simulink model "adaptive_control"  (R2019a)
settings: Solver=ode3  StartTime=0.0  StopTime=15  FixedStep=.002  RelTol=1e-3  EnableMultiTasking=on
settings Model: ExtModeTrigDuration=10000  Creator=smascaro  LastModifiedBy=hoops
settings SolverCC: PositivePriorityOrder=on
settings DataIOCC: SaveFormat=Array  SignalLoggingSaveFormat=ModelDataLogs  SaveOutput=off  SaveTime=off  ReturnWorkspaceOutputs=off
settings OptimizationCC: ExpressionDepthLimit=2147483647  InitFltsAndDblsToZero=on  LifeSpan=inf
settings DebuggingCC: SaveWithParameterizedLinksMsg=none  UnderspecifiedInitializationDetection=Classic  MergeDetectMultiDrivingBlocksExec=none  SignalResolutionControl=TryResolveAllWithWarning  SolverPrmCheckMsg=warning  MultiTaskDSMMsg=warning  MultiTaskCondExecSysMsg=none  FcnCallInpInsideContextMsg=warning  AllowSymbolicDim=off  StateNameClashWarn=warning  SFUnexpectedBacktrackingDiag=warning  SFNoUnconditionalDefaultTransitionDiag=warning  SFExecutionAtInitializationDiag=none  ArithmeticOperatorsInVariantConditions=warning
settings HardwareCC: ProdBitPerPointer=32  ProdBitPerSizeT=32  ProdBitPerPtrDiffT=32  ProdLargestAtomicFloat=None  ProdIntDivRoundTo=Undefined  ProdEndianess=Unspecified  ProdWordSize=32  ProdHWDeviceType=32-bit Generic  TargetBitPerPointer=64  TargetBitPerSizeT=64  TargetBitPerPtrDiffT=64  TargetLongLongMode=on  TargetIntDivRoundTo=Zero  TargetEndianess=LittleEndian  TargetWordSize=64  TargetHWDeviceType=MATLAB Host
settings ModelReferenceCC: PropagateSignalLabelsOutOfModel=off
settings SFSimCC: SimUseLocalCustomCode=off  SimParseCustomCode=off
settings RTWCC: SystemTargetFile=quarc_windows.tlc  TemplateMakefile=quarc_default_tmf  Description=QUARC Win32 Target  RTWUseLocalCustomCode=off
settings CodeAppCC: StateflowObjectComments=on
settings STFCustomTargetCC: TargetPreCompLibLocation=C:\PROGRA~3\QUARC\lib\2015b\windows\release  GeneratePreprocessorConditionals=Disable all  CPPClassGenCompliant=on  SystemTargetFile=quarc_windows.tlc
settings GRTTargetCC: TargetPreCompLibLocation=C:\PROGRA~3\QUARC\lib\2015b\windows\release  TargetLangStandard=C89/C90 (ANSI)  ParMdlRefBuildCompliant=off  CompOptLevelCompliant=off  ConcurrentExecutionCompliant=off  GeneratePreprocessorConditionals=Disable all  CombineOutputUpdateFcns=off  MatFileLogging=off  GRTInterface=on  UseToolchainInfoCompliant=off  ExtMode=on  ExtModeMexFile=quarc_comm
settings ConfigComp: CovMetricSettings=dw  CovHtmlReporting=on  CovSaveCumulativeToWorkspaceVar=on  CovSaveSingleToWorkspaceVar=on  CovExternalEMLEnable=off

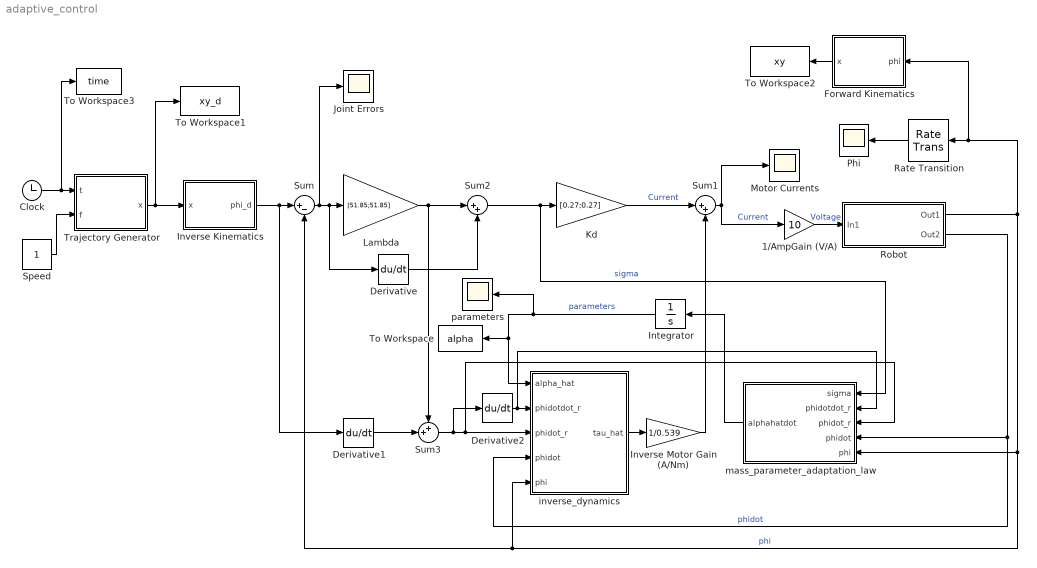
== system adaptive_control ==
  1/AmpGain (V/A) : Gain  Gain=10
  Clock : Clock
  Derivative : Derivative
  Derivative1 : Derivative
  Derivative2 : Derivative
  Forward Kinematics : MATLAB Function  TreatAsAtomicUnit=on
  Integrator : Integrator  InitialCondition=[0.001; 0.001; 0.001; 0.001]
  Inverse Kinematics : MATLAB Function  TreatAsAtomicUnit=on
  Inverse Motor Gain (A/Nm) : Gain  Gain=1/0.539
  Joint Errors : Scope
  Kd : Gain  Gain=[0.27;0.27]
  Lambda : Gain  Gain=[51.85;51.85]
  Motor Currents : Scope
  Phi : Scope
      settings: AttributesFormatString=SampleTime =%<SampleTime>
  Rate Transition : RateTransition  OutPortSampleTimeOpt=Inherit  OutPortSampleTimeMultiple=10  OutPortSampleTime=0.05
  Robot : Subsystem
      mask Display: disp('Manipulator')
  Speed : Constant
      settings: AttributesFormatString=(circles/sec)
  Sum : Sum  Inputs=|+-
  Sum1 : Sum  Inputs=|++
  Sum2 : Sum  Inputs=|++
  Sum3 : Sum  Inputs=++|
  To Workspace : ToWorkspace  VariableName=alpha  SampleTime=-1
  To Workspace1 : ToWorkspace  VariableName=xy_d  SampleTime=-1
  To Workspace2 : ToWorkspace  VariableName=xy  SampleTime=-1
  To Workspace3 : ToWorkspace  VariableName=time  SampleTime=-1
  Trajectory Generator : MATLAB Function  TreatAsAtomicUnit=on
  inverse_dynamics : MATLAB Function  TreatAsAtomicUnit=on
  "mass_parameter_adaptation_law " : MATLAB Function  TreatAsAtomicUnit=on
  parameters : Scope
  wires:
  Robot/1(Out1) -> Forward Kinematics/1(phi), Rate Transition/1, "mass_parameter_adaptation_law "/5(phi), inverse_dynamics/5(phi), Sum/2  "phi"
  Inverse Kinematics/1(phi_d) -> Derivative1/1, Sum/1
  Trajectory Generator/1(x) -> Inverse Kinematics/1(x), To Workspace1/1
  Forward Kinematics/1(x) -> To Workspace2/1
  Clock/1 -> To Workspace3/1, Trajectory Generator/1(t)
  Speed/1 -> Trajectory Generator/2(f)
  1/AmpGain (V/A)/1 -> Robot/1(In1)  "Voltage"
  Sum/1 -> Derivative/1, Lambda/1, Joint Errors/1
  Sum1/1 -> 1/AmpGain (V/A)/1, Motor Currents/1  "Current"
  Rate Transition/1 -> Phi/1
  Kd/1 -> Sum1/1  "Current"
  inverse_dynamics/1(tau_hat) -> Inverse Motor Gain (A/Nm)/1
  Inverse Motor Gain (A/Nm)/1 -> Sum1/2
  Lambda/1 -> Sum2/1, Sum3/1
  Derivative/1 -> Sum2/2
  Derivative1/1 -> Sum3/2
  Sum2/1 -> "mass_parameter_adaptation_law "/1(sigma), Kd/1  "sigma"
  Sum3/1 -> Derivative2/1, "mass_parameter_adaptation_law "/3(phidot_r), inverse_dynamics/3(phidot_r)
  Derivative2/1 -> "mass_parameter_adaptation_law "/2(phidotdot_r), inverse_dynamics/2(phidotdot_r)
  Robot/2(Out2) -> inverse_dynamics/4(phidot), "mass_parameter_adaptation_law "/4(phidot)  "phidot"
  "mass_parameter_adaptation_law "/1(alphahatdot) -> Integrator/1
  Integrator/1 -> parameters/1, To Workspace/1, inverse_dynamics/1(alpha_hat)  "parameters"

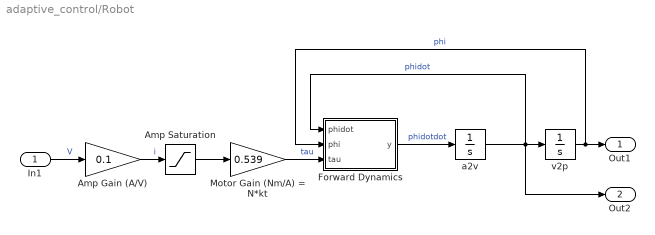
== system adaptive_control/Robot ==
  In1 : Inport
  Amp Saturation : Saturate  UpperLimit=1  LowerLimit=-1  ZeroCross=off
  Amp Gain (A/V) : Gain  Gain=0.1
  Forward Dynamics : MATLAB Function  TreatAsAtomicUnit=on
  Motor Gain (Nm/A) = N*kt : Gain  Gain=0.539
  a2v : Integrator
  v2p : Integrator  InitialCondition=[1.1934;-0.2661]
  Out1 : Outport
  Out2 : Outport  Port=2
  wires:
  Forward Dynamics/1(y) -> a2v/1  "phidotdot"
  a2v/1 -> v2p/1, Out2/1, Forward Dynamics/1(phidot)  "phidot"
  v2p/1 -> Out1/1, Forward Dynamics/2(phi)  "phi"
  In1/1 -> Amp Gain (A/V)/1  "V"
  Motor Gain (Nm/A) = N*kt/1 -> Forward Dynamics/3(tau)  "tau"
  Amp Saturation/1 -> Motor Gain (Nm/A) = N*kt/1
  Amp Gain (A/V)/1 -> Amp Saturation/1  "i"

== matlab function adaptive_control/Inverse Kinematics ==
  settings: fimath=|
      | fimath(...
      | 'RoundMode', 'floor',...
      | 'OverflowMode', 'wrap',...
      | 'ProductMode', 'KeepLSB', 'ProductWordLength', 32,...
      | 'SumMode', 'KeepLSB', 'SumWordLength', 32,...
      | 'CastBeforeSum', false)
  data: x input; phi_d output
function phi_d = fcn(x)
% This block supports an embeddable subset of the MATLAB language.
% See the help menu for details. 
a1=0.15;
a2=0.15;
Jt = [1 0;-1 1]; % transmission Jacobian for belt drive

theta = [0;0];
theta(2) = -2*atan(sqrt(((a1+a2)^2-(x(1)^2+x(2)^2))/((x(1)^2+x(2)^2)-(a1-a2)^2)));
theta(1) = atan2(x(2),x(1))-atan2(a2*sin(theta(2)),a1+a2*cos(theta(2)));

phi_d = inv(Jt)*theta;

== matlab function adaptive_control/Robot/Forward Dynamics ==
  settings: fimath=|
      | fimath(...
      | 'RoundMode', 'floor',...
      | 'OverflowMode', 'wrap',...
      | 'ProductMode', 'KeepLSB', 'ProductWordLength', 32,...
      | 'SumMode', 'KeepLSB', 'SumWordLength', 32,...
      | 'CastBeforeSum', false)
  data: phidot input double size=2; phi input double size=2; y output double size=2; tau input size=2
function y = fcn(phidot,phi,tau)
% This block supports an embeddable subset of the MATLAB language.
% See the help menu for details. 

a1 = 0.15;  % link 1 length
a2 = 0.15;  % link 2 length
m1 = 0.092;  % link 1 mass  
m2 = 0.077; % link 2 mas
r01 = 0.062; % link 1 center of mass
r12 = 0.036; % link 2 COM
I1 = 0.64e-3;  % link 1 inertia
I2 = 0.30e-3;  % link 2 inertia
Jm1 = 0.65e-6; % motor inertias
Jm2 = 0.65e-6;
b1 = 3.1e-6; % viscous damping constants
b2 = 3.1e-6;
c1 = 0.0001; % coulomb friction constants
c2 = 0.0001;
g = 9.8; % gravitational constant
N1 = 70; % gear ratios
N2 = 70;

H11 = N1^2*Jm1 + I1 + m2*a1^2;
H12 = a1*r12*m2*cos(phi(2)-phi(1));
H21 = H12;
H22 = N2^2*Jm2 + I2;
h = a1*r12*m2*sin(phi(2)-phi(1));
G1 = (r01*m1+a1*m2)*g*cos(phi(1));
G2 = r12*m2*g*cos(phi(2));
F1 = N1^2*b1*phidot(1) + N1*c1*sign(phidot(1));
F2 = N2^2*b2*phidot(2) + N2*c2*sign(phidot(2));

H = [H11 H12; H21 H22]; % inertia matrix
V = [0 -h ;h 0]*[phidot(1)^2;phidot(2)^2]; % centripetal torques
G = [G1;G2]; % gravity torques
F = [F1;F2]; % frictional torques

y = inv(H)*(tau - V - G - F); % y=phidotdot

== matlab function adaptive_control/Forward Kinematics ==
  settings: fimath=|
      | fimath(...
      | 'RoundMode', 'floor',...
      | 'OverflowMode', 'wrap',...
      | 'ProductMode', 'KeepLSB', 'ProductWordLength', 32,...
      | 'SumMode', 'KeepLSB', 'SumWordLength', 32,...
      | 'CastBeforeSum', false)
  data: x output; phi input
function x = fcn(phi)
% This block supports an embeddable subset of the MATLAB language.
% See the help menu for details. 

a1=0.15;
a2=0.15;
x = [0;0];
x(1) = a1*cos(phi(1))+a2*cos(phi(2));
x(2) = a1*sin(phi(1))+a2*sin(phi(2));

== matlab function adaptive_control/inverse_dynamics ==
  settings: fimath=|
      | fimath(...
      | 'RoundMode', 'floor',...
      | 'OverflowMode', 'wrap',...
      | 'ProductMode', 'KeepLSB', 'ProductWordLength', 32,...
      | 'SumMode', 'KeepLSB', 'SumWordLength', 32,...
      | 'CastBeforeSum', false)
  data: alpha_hat input size=4; phidotdot_r input; phidot_r input; phidot input double size=2; phi input double size=2; tau_hat output double size=2
function tau_hat = fcn(alpha_hat,phidotdot_r,phidot_r,phidot,phi)
% This block supports an embeddable subset of the MATLAB language.
% See the help menu for details. 

a1 = 0.15;  % link 1 length
a2 = 0.15;  % link 2 length
b1 = 3.1e-6; % viscous damping constants
b2 = 3.1e-6;
c1 = 0.0001; % coulomb friction constants
c2 = 0.0001;
g = 9.8; % gravitational constant
N1 = 70; % gear ratios
N2 = 70;

F1 = N1^2*b1*phidot(1) + N1*c1*sign(phidot(1));
F2 = N2^2*b2*phidot(2) + N2*c2*sign(phidot(2));

F = [F1;F2]; % frictional torques

Y11 = phidotdot_r(1);
Y12 = a1*cos(phi(2)-phi(1))*phidotdot_r(2) - a1*sin(phi(2)-phi(1))*phidot(2)*phidot_r(2);
Y13 = g*cos(phi(1));
Y14 = 0;
Y21 = 0;
Y22 = a1*cos(phi(2)-phi(1))*phidotdot_r(1) + a1*sin(phi(2)-phi(1))*phidot(1)*phidot_r(1) + g*cos(phi(2));
Y23 = 0;
Y24 = phidotdot_r(2);

Y = [Y11 Y12 Y13 Y14; Y21 Y22 Y23 Y24];


tau_hat = Y*alpha_hat + F;

== matlab function adaptive_control/mass_parameter_adaptation_law  ==
  data: sigma input; alphahatdot output; phidotdot_r input; phidot_r input; phidot input; phi input
function alphahatdot = fcn(sigma,phidotdot_r,phidot_r,phidot,phi)
% This block supports an embeddable subset of the MATLAB language.
% See the help menu for details. 

a1 = 0.15;  % link 1 length
a2 = 0.15;  % link 2 length

g = 9.8; % gravitational constant

Y11 = phidotdot_r(1);
Y12 = a1*cos(phi(2)-phi(1))*phidotdot_r(2) - a1*sin(phi(2)-phi(1))*phidot(2)*phidot_r(2);
Y13 = g*cos(phi(1));
Y14 = 0;
Y21 = 0;
Y22 = a1*cos(phi(2)-phi(1))*phidotdot_r(1) + a1*sin(phi(2)-phi(1))*phidot(1)*phidot_r(1) + g*cos(phi(2));
Y23 = 0;
Y24 = phidotdot_r(2);

Y = [Y11 Y12 Y13 Y14; Y21 Y22 Y23 Y24];

gamma_val = 15  ;
gamma = [gamma_val 0 0 0; 0 gamma_val 0 0; 0 0 gamma_val 0; 0 0 0 gamma_val];

alphahatdot = inv(gamma) * transpose(Y) * sigma;

== matlab function adaptive_control/Trajectory Generator ==
  settings: fimath=|
      | fimath(...
      | 'RoundMode', 'floor',...
      | 'OverflowMode', 'wrap',...
      | 'ProductMode', 'KeepLSB', 'ProductWordLength', 32,...
      | 'SumMode', 'KeepLSB', 'SumWordLength', 32,...
      | 'CastBeforeSum', false)
  data: x output; t input; f input
function x = fcn(t,f)
% This block supports an embeddable subset of the MATLAB language.
% See the help menu for details. 
x = [0;0];

if t<0.5  % accelerate into circling trajectory
    x(1) = 0.075*cos(2*pi*f*t^2) + 0.125;
    x(2) = 0.075*sin(2*pi*f*t^2) + 0.1;
else  % constant speed circling of radius 0.075 about x=[0.125,0.1]
    x(1) = 0.075*cos(2*pi*f*(t-0.25)) + 0.125;
    x(2) = 0.075*sin(2*pi*f*(t-0.25)) + 0.1;
end
